simulink model "helloWorld"  (R2024a)
settings: Solver=FixedStepAuto  StartTime=0.0  StopTime=inf  RelTol=1e-3
undefined symbols (not defined in the file): Payload
libraries: uavmavlinklib x8, simulink_extras x3, aerolibanimutils x1, instrumentlib x1
settings Model: Creator=Alireza  LastModifiedBy=user
settings RTWCC: GPUComputeCapability=3.5

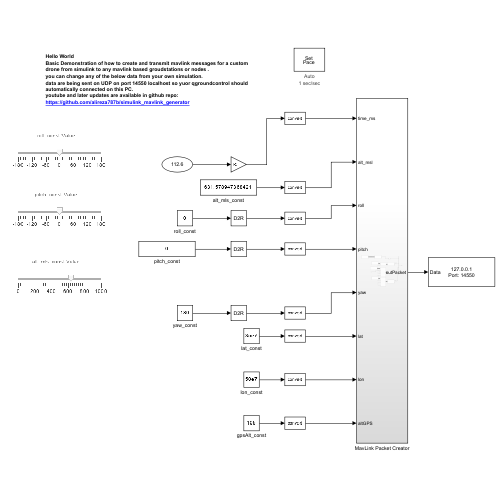
[thumbnail: Simulink's stored preview of the top-level diagram]
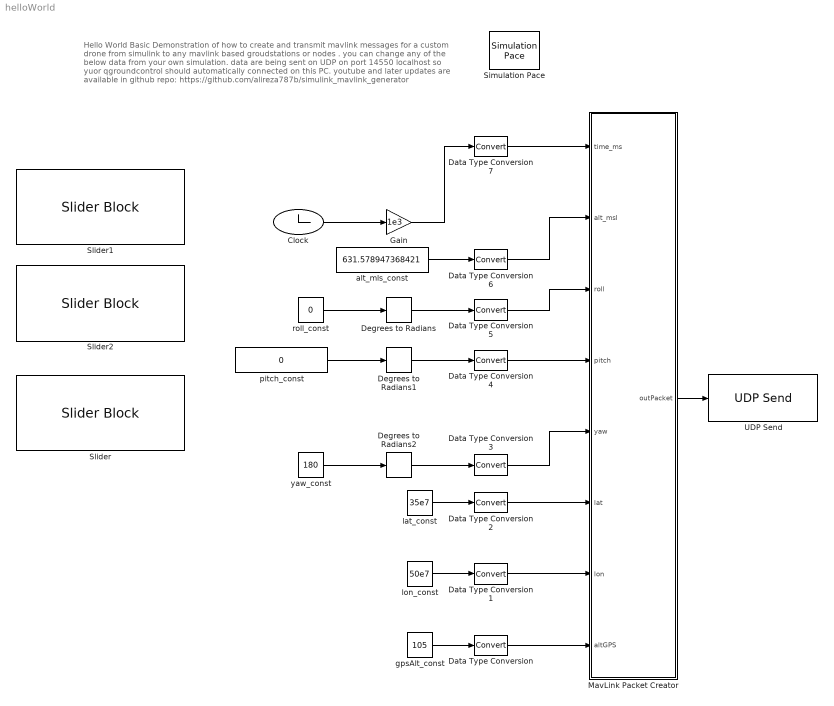
== system helloWorld ==
  note: Hello World
      | Basic Demonstration of how to create and transmit mavlink messages for a custom drone from simulink to any mavlink based groudstations or nodes .
      | you can change any of the below data from your own simulation.
      | data are being sent on UDP on port 14550 localhost so yuor qgroundcontrol should automatically connected on this PC.
      | youtube and later updates are available in github repo:
      | https://github.com/alireza787b/simulink_mavlink_generator
  Clock : Clock
      settings: Decimation=3
  Data Type Conversion{,1..7} (8 alike) : DataTypeConversion  SaturateOnIntegerOverflow=off  RndMeth=Floor
  Degrees to Radians : simulink_extras/Transformations/Degrees to Radians
  Degrees to Radians1 : simulink_extras/Transformations/Degrees to Radians
  Degrees to Radians2 : simulink_extras/Transformations/Degrees to Radians
  Gain : Gain  Gain=1e3
  MavLink Packet Creator : Subsystem
  Simulation Pace : aerolibanimutils/Simulation Pace  SimulationPace=1  SleepMode=Auto  OutputPaceError=off  SampleTime=-1
  Slider : SliderBlock  ScaleMax=1000
  Slider1 : SliderBlock  ScaleMin=-180  ScaleMax=180
  Slider2 : SliderBlock  ScaleMin=-180  ScaleMax=180
  UDP Send : instrumentlib/UDP Send  Host=127.0.0.1  Port=14550  LocalAddress=127.0.0.1  LocalPort=-1  EnablePortSharing=off  OutputDatagramPacketSize=512  ByteOrder=big-endian  EnableBlockingMode=on  SimulateUsing=Interpreted execution
  alt_mls_const : Constant  Value=631.578947368421  SampleTime=-1
  gpsAlt_const : Constant  Value=105  SampleTime=-1
  lat_const : Constant  Value=35e7  SampleTime=-1
  lon_const : Constant  Value=50e7  SampleTime=-1
  pitch_const : Constant  Value=0  SampleTime=-1
  roll_const : Constant  Value=0  SampleTime=-1
  yaw_const : Constant  Value=180  SampleTime=-1
  wires:
  lat_const/1 -> Data Type Conversion2/1
  Clock/1 -> Gain/1
  Data Type Conversion4/1 -> MavLink Packet Creator/4(pitch)
  Data Type Conversion6/1 -> MavLink Packet Creator/2(alt_msl)
  roll_const/1 -> Degrees to Radians/1
  yaw_const/1 -> Degrees to Radians2/1
  Degrees to Radians1/1 -> Data Type Conversion4/1
  alt_mls_const/1 -> Data Type Conversion6/1
  pitch_const/1 -> Degrees to Radians1/1
  Gain/1 -> Data Type Conversion7/1
  Degrees to Radians/1 -> Data Type Conversion5/1
  Degrees to Radians2/1 -> Data Type Conversion3/1
  lon_const/1 -> Data Type Conversion1/1
  gpsAlt_const/1 -> Data Type Conversion/1
  MavLink Packet Creator/1(outPacket) -> UDP Send/1
  Data Type Conversion7/1 -> MavLink Packet Creator/1(time_ms)
  Data Type Conversion5/1 -> MavLink Packet Creator/3(roll)
  Data Type Conversion1/1 -> MavLink Packet Creator/7(lon)
  Data Type Conversion3/1 -> MavLink Packet Creator/5(yaw)
  Data Type Conversion/1 -> MavLink Packet Creator/8(altGPS)
  Data Type Conversion2/1 -> MavLink Packet Creator/6(lat)

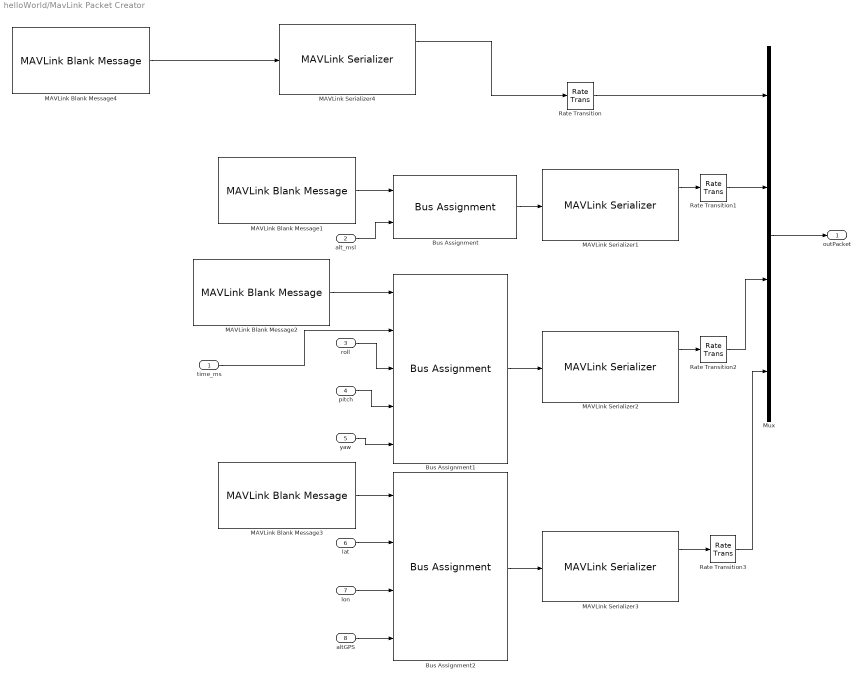
== system helloWorld/MavLink Packet Creator ==
  time_ms : Inport
  alt_msl : Inport  Port=2
  roll : Inport  Port=3
  pitch : Inport  Port=4
  yaw : Inport  Port=5
  lat : Inport  Port=6
  lon : Inport  Port=7
  altGPS : Inport  Port=8
  Bus Assignment : BusAssignment  AssignedSignals=Payload.altitude_amsl
  Bus Assignment1 : BusAssignment  AssignedSignals=Payload.time_boot_ms,Payload.roll,Payload.pitch,Payload.yaw
  Bus Assignment2 : BusAssignment  AssignedSignals=Payload.lat,Payload.lon,Payload.alt
  MAVLink Blank Message1 : uavmavlinklib/MAVLink Blank Message  dialectSource=Select from standard MAVLink dialects  dialect=common.xml  dialectCustom=common.xml  version=2  messageType=ALTITUDE  SystemID=2  ComponentID=1  SampleTime=-1
  MAVLink Blank Message2 : uavmavlinklib/MAVLink Blank Message  dialectSource=Select from standard MAVLink dialects  dialect=common.xml  dialectCustom=common.xml  version=2  messageType=ATTITUDE  SystemID=2  ComponentID=1  SampleTime=-1
  MAVLink Blank Message3 : uavmavlinklib/MAVLink Blank Message  dialectSource=Select from standard MAVLink dialects  dialect=common.xml  dialectCustom=common.xml  version=2  messageType=GLOBAL_POSITION_INT  SystemID=2  ComponentID=1  SampleTime=-1
  MAVLink Blank Message4 : uavmavlinklib/MAVLink Blank Message  dialectSource=Select from standard MAVLink dialects  dialect=common.xml  dialectCustom=common.xml  version=2  messageType=HEARTBEAT  SystemID=2  ComponentID=1  SampleTime=-1
  MAVLink Serializer1 : uavmavlinklib/MAVLink Serializer  dialectSource=Select from standard MAVLink dialects  dialect=common.xml  dialectCustom=common.xml  version=2  messageType=ALTITUDE
  MAVLink Serializer2 : uavmavlinklib/MAVLink Serializer  dialectSource=Select from standard MAVLink dialects  dialect=common.xml  dialectCustom=common.xml  version=2  messageType=ATTITUDE
  MAVLink Serializer3 : uavmavlinklib/MAVLink Serializer  dialectSource=Select from standard MAVLink dialects  dialect=common.xml  dialectCustom=common.xml  version=2  messageType=GLOBAL_POSITION_INT
  MAVLink Serializer4 : uavmavlinklib/MAVLink Serializer  dialectSource=Select from standard MAVLink dialects  dialect=common.xml  dialectCustom=common.xml  version=2  messageType=HEARTBEAT
  Mux : Mux
  Rate Transition{,1..3} (4 alike) : RateTransition
  outPacket : Outport
  wires:
  yaw/1 -> Bus Assignment1/5
  roll/1 -> Bus Assignment1/3
  MAVLink Blank Message3/1 -> Bus Assignment2/1
  alt_msl/1 -> Bus Assignment/2
  MAVLink Blank Message1/1 -> Bus Assignment/1
  MAVLink Blank Message2/1 -> Bus Assignment1/1
  pitch/1 -> Bus Assignment1/4
  lat/1 -> Bus Assignment2/2
  lon/1 -> Bus Assignment2/3
  altGPS/1 -> Bus Assignment2/4
  Mux/1 -> outPacket/1
  Bus Assignment/1 -> MAVLink Serializer1/1
  Bus Assignment1/1 -> MAVLink Serializer2/1
  Bus Assignment2/1 -> MAVLink Serializer3/1
  MAVLink Serializer1/1 -> Rate Transition1/1
  MAVLink Serializer2/1 -> Rate Transition2/1
  MAVLink Serializer3/1 -> Rate Transition3/1
  Rate Transition/1 -> Mux/1
  Rate Transition1/1 -> Mux/2
  Rate Transition2/1 -> Mux/3
  Rate Transition3/1 -> Mux/4
  MAVLink Blank Message4/1 -> MAVLink Serializer4/1
  MAVLink Serializer4/1 -> Rate Transition/1
  time_ms/1 -> Bus Assignment1/2
